simulink model "image_based_tracking"  (R2015b)
settings: Solver=ode45  StartTime=0.0  StopTime=50  RelTol=1e-3
InitFcn:
  | param
undefined symbols (not defined in the file or in its folder): ctrl, P
settings Model: Creator=beard  LastModifiedBy=magiccjae
settings DataIOCC: SaveFormat=Array  SignalLoggingSaveFormat=ModelDataLogs
settings OptimizationCC: ExpressionDepthLimit=2147483647  InitFltsAndDblsToZero=on
settings DebuggingCC: UnderspecifiedInitializationDetection=Classic  MergeDetectMultiDrivingBlocksExec=none  SolverPrmCheckMsg=warning  FcnCallInpInsideContextMsg=UseLocalSettings  StateNameClashWarn=warning
settings HardwareCC: ProdBitPerPointer=32  ProdLargestAtomicFloat=None  ProdIntDivRoundTo=Undefined  ProdEndianess=Unspecified  ProdWordSize=32  ProdHWDeviceType=32-bit Generic
settings GRTTargetCC: GeneratePreprocessorConditionals=Disable all  CombineOutputUpdateFcns=off  GRTInterface=on
settings ConfigComp: CovModelRefEnable=Off

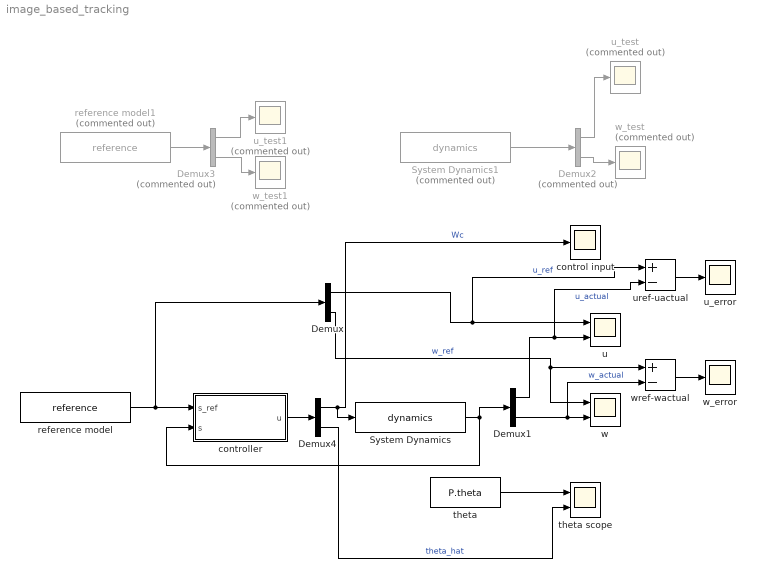
== system image_based_tracking ==
  Demux : Demux  Outputs=2
  Demux1 : Demux  Outputs=2
  Demux2 : Demux  Commented=on  Outputs=2
  Demux3 : Demux  Commented=on  Outputs=2
  Demux4 : Demux  Outputs=[3 1]
  System Dynamics : S-Function  FunctionName=dynamics  Parameters=P  SFunctionDeploymentMode=off  EnableBusSupport=off
  System Dynamics1 : S-Function  Commented=on  FunctionName=dynamics  Parameters=P  SFunctionDeploymentMode=off  EnableBusSupport=off
  control input : Scope
  controller : Subsystem
  reference model : S-Function  FunctionName=reference  Parameters=P  SFunctionDeploymentMode=off  EnableBusSupport=off
  reference model1 : S-Function  Commented=on  FunctionName=reference  Parameters=P  SFunctionDeploymentMode=off  EnableBusSupport=off
  theta : Constant  Value=P.theta
  theta scope : Scope  NumInputPorts=2
  u : Scope  NumInputPorts=2
  u_error : Scope
  u_test : Scope  Commented=on
  u_test1 : Scope  Commented=on
  uref-uactual : Sum  Inputs=+-
  w : Scope  NumInputPorts=2
  w_error : Scope
  w_test : Scope  Commented=on
  w_test1 : Scope  Commented=on
  wref-wactual : Sum  Inputs=+-
  wires:
  reference model/1 -> Demux/1, controller/1(s_ref)
  System Dynamics/1 -> controller/2(s), Demux1/1
  Demux1/2 -> wref-wactual/2, w/2  "w_actual"
  Demux/1 -> uref-uactual/1, u/1  "u_ref"
  Demux/2 -> wref-wactual/1, w/1  "w_ref"
  Demux1/1 -> uref-uactual/2, u/2  "u_actual"
  System Dynamics1/1 -> Demux2/1
  Demux2/1 -> u_test/1
  Demux2/2 -> w_test/1
  Demux3/1 -> u_test1/1
  Demux3/2 -> w_test1/1
  reference model1/1 -> Demux3/1
  controller/1(u) -> Demux4/1
  Demux4/1 -> control input/1, System Dynamics/1  "Wc"
  uref-uactual/1 -> u_error/1
  wref-wactual/1 -> w_error/1
  Demux4/2 -> theta scope/2  "theta_hat"
  theta/1 -> theta scope/1

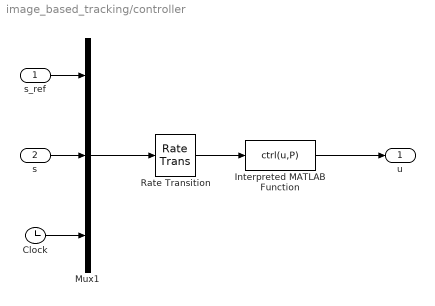
== system image_based_tracking/controller ==
  s_ref : Inport
  s : Inport  Port=2
  Clock : Clock
  Interpreted MATLAB Function : MATLABFcn  MATLABFcn=ctrl(u,P)  OutputDimensions=4
  Mux1 : Mux  Inputs=3
  Rate Transition : RateTransition  OutPortSampleTime=P.Ts
  u : Outport
  wires:
  Mux1/1 -> Rate Transition/1
  s_ref/1 -> Mux1/1
  Interpreted MATLAB Function/1 -> u/1
  Rate Transition/1 -> Interpreted MATLAB Function/1
  s/1 -> Mux1/2
  Clock/1 -> Mux1/3
